simulink model "P413_3_model"  (R2021a)
settings: Solver=VariableStepAuto  StartTime=0.0  StopTime=tspan(end)  RelTol=1e-3
values from neighbouring files (symbols this model uses):
  AR = params(1).Value    [P413_3_clima.m]
  beta = params(1).Value    [P413_3_clima.m]
  gamma = params(2).Value    [P413_3_clima.m]
  Tmax = 273.15 + 20    (= 293.15)    [P413_3_clima.m]
  Tstart = 273.15 + 10    (= 283.15)    [P413_3_clima.m]
libraries: HORTISIM x6
settings Model: OrderedModelArguments=off  Creator=djoroya  LastModifiedBy=djoroya
settings DataIOCC: ExternalInput=tp3276776d_8610_4451_82d6_0aeb35eee2de(1)  OutputOption=AdditionalOutputTimes  OutputTimes=SDO_OutputTimes  ReturnWorkspaceOutputsName=SDOSimTest_Log

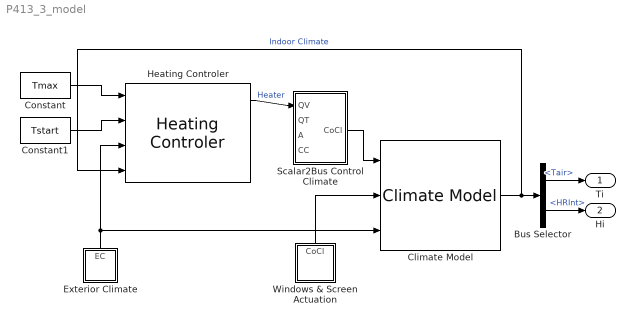
== system P413_3_model ==
  Bus Selector : BusSelector  OutputSignals=Temp.Tair,Gas.HRInt
  Climate Model : HORTISIM/Climate/Models/Climate Model  params=p_ic  x0=x0_ic
      settings: SourceProductName=Horti Simulator
  Constant : Constant  Value=Tmax
  Constant1 : Constant  Value=Tstart
  Exterior Climate : Subsystem
  Heating Controler : HORTISIM/Climate/Controls/Heating Controler  params=HP  x0=x0_H
      settings: SourceProductName=Horti Simulator
  Scalar2Bus Control Climate : Subsystem
  Windows & Screen Actuation : Subsystem
  Ti : Outport
  Hi : Outport  Port=2
  wires:
  Exterior Climate/1(EC) -> Climate Model/3, Heating Controler/3
  Climate Model/1 -> Heating Controler/4, Bus Selector/1  "Indoor Climate"
  Bus Selector/1 -> Ti/1  "<Tair>"
  Windows & Screen Actuation/1(CoCl) -> Climate Model/2
  Bus Selector/2 -> Hi/1  "<HRInt>"
  Scalar2Bus Control Climate/1(CoCl) -> Climate Model/1
  Heating Controler/1 -> Scalar2Bus Control Climate/1(QV)  "Heater"
  Constant/1 -> Heating Controler/1
  Constant1/1 -> Heating Controler/2

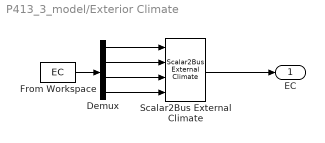
== system P413_3_model/Exterior Climate ==
  Demux : Demux
  From Workspace : FromWorkspace  VariableName=EC
  Scalar2Bus External Climate : HORTISIM/Other  Functions/Scalar2Bus External Climate  SystemSampleTime=-1  VariantActivationTime=update diagram  Latency=0  AutoFrameSizeCalculation=off
      settings: SourceProductName=Horti Simulator
  EC : Outport
  wires:
  Demux/3 -> Scalar2Bus External Climate/3
  Demux/2 -> Scalar2Bus External Climate/2
  Scalar2Bus External Climate/1 -> EC/1
  Demux/1 -> Scalar2Bus External Climate/1
  Demux/4 -> Scalar2Bus External Climate/4
  From Workspace/1 -> Demux/1

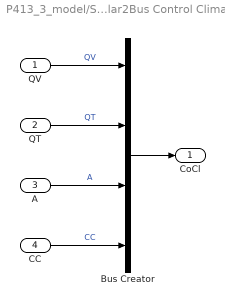
== system P413_3_model/Scalar2Bus Control Climate ==
  QV : Inport
  QT : Inport  Port=2
  A : Inport  Port=3
  CC : Inport  Port=4
  Bus Creator : BusCreator  Inputs=4
  CoCl : Outport
  wires:
  A/1 -> Bus Creator/3  "A"
  CC/1 -> Bus Creator/4  "CC"
  QV/1 -> Bus Creator/1  "QV"
  Bus Creator/1 -> CoCl/1
  QT/1 -> Bus Creator/2  "QT"

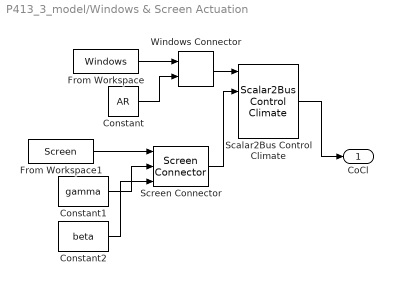
== system P413_3_model/Windows & Screen Actuation ==
  Constant : Constant  Value=AR
  Constant1 : Constant  Value=gamma
  Constant2 : Constant  Value=beta
  From Workspace : FromWorkspace  VariableName=Windows
  From Workspace1 : FromWorkspace  VariableName=Screen
  Scalar2Bus Control Climate : HORTISIM/Other  Functions/Scalar2Bus  Control Climate  SystemSampleTime=-1  VariantActivationTime=update diagram  Latency=0  AutoFrameSizeCalculation=off
      settings: SourceProductName=Horti Simulator
  Screen Connector : HORTISIM/Other  Functions/Screen Connector  SystemSampleTime=-1  VariantActivationTime=update diagram  Latency=0  AutoFrameSizeCalculation=off
      settings: SourceProductName=Horti Simulator
  Windows Connector : HORTISIM/Other  Functions/Windows Connector  SystemSampleTime=-1  VariantActivationTime=update diagram  Latency=0  AutoFrameSizeCalculation=off
      settings: SourceProductName=Horti Simulator
  CoCl : Outport
  wires:
  Screen Connector/1 -> Scalar2Bus Control Climate/2
  Scalar2Bus Control Climate/1 -> CoCl/1
  From Workspace1/1 -> Screen Connector/1
  Constant/1 -> Windows Connector/2
  Windows Connector/1 -> Scalar2Bus Control Climate/1
  Constant1/1 -> Screen Connector/2
  From Workspace/1 -> Windows Connector/1
  Constant2/1 -> Screen Connector/3
